simulink model "p4"  (R2015a)
settings: Solver=ode45  StartTime=0.0  StopTime=10.0  RelTol=1e-3
undefined symbols (not defined in the file or in its folder): K
settings Model: Creator=jgutierr  LastModifiedBy=vdrouinv

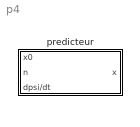
== system p4 ==
  predicteur : Subsystem  TreatAsAtomicUnit=on

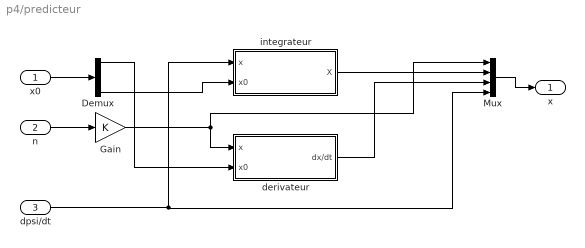
== system p4/predicteur ==
  x0 : Inport
  n : Inport  Port=2
  dpsi/dt : Inport  Port=3
  Demux : Demux
  Gain : Gain  Gain=K
  Mux : Mux
  derivateur : Subsystem  TreatAsAtomicUnit=on
  integrateur : Subsystem  TreatAsAtomicUnit=on
  x : Outport
  wires:
  x0/1 -> Demux/1
  dpsi/dt/1 -> integrateur/1(x), Mux/4
  Demux/4 -> integrateur/2(x0)
  Demux/1 -> derivateur/2(x0)
  n/1 -> Gain/1
  Gain/1 -> Mux/1, derivateur/1(x)
  Mux/1 -> x/1
  integrateur/1(X) -> Mux/2
  derivateur/1(dx/dt) -> Mux/3

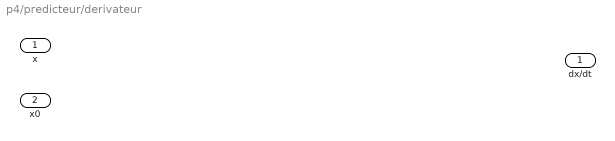
== system p4/predicteur/derivateur ==
  x : Inport
  x0 : Inport  Port=2
  dx/dt : Outport

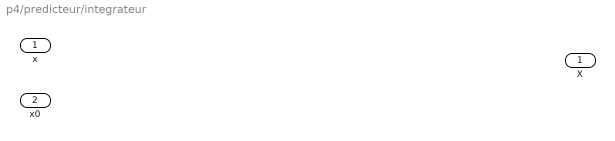
== system p4/predicteur/integrateur ==
  x : Inport
  x0 : Inport  Port=2
  X : Outport
